simulink model "QMF_lattice"  (Simulink 7.9)
settings: Solver=ode45  StartTime=0.0  StopTime=10  RelTol=1e-3
undefined symbols (not defined in the file or in its folder): dfilt, Fs, get, sided, Two
libraries: dspsigops x6, dsparch4 x4, dspsnks4 x4, dspvision x1, simulink x1, dspsrcs4 x1
settings Model: Creator=Arun  LastModifiedBy=Arun

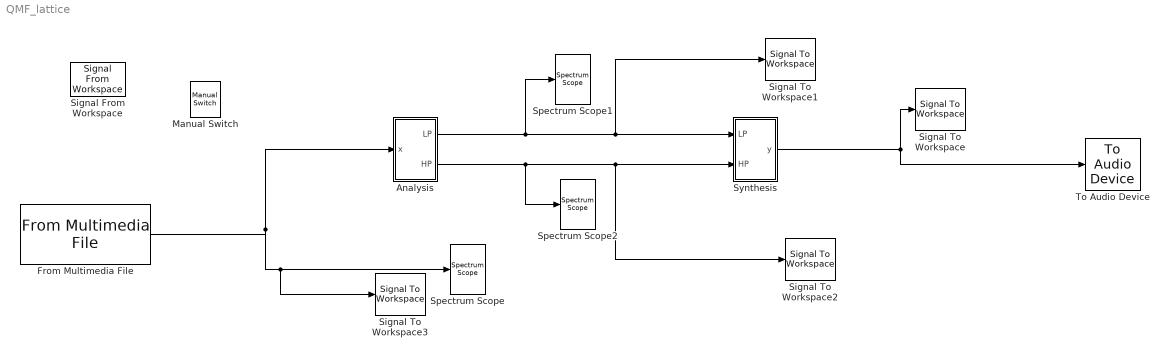
== system QMF_lattice ==
  Analysis : Subsystem
  From Multimedia File : dspvision/From Multimedia File  inputFilename=I:\Documents and Settings\Arun\My Documents\MATLAB\QMF\CRASH.WAV  loop=on  numPlays=inf  outputStreams=Audio only  videoDataType=single  audioDataType=int16  inheritSampleTime=on  userDefinedSampleTime=1/30  noAudioOutput=off  isIntensityVideo=off  fourcc=RGB  colorVideoFormat=Separate color signals  outputEOF=off  dataOrg=Column-major  audioFrameSize=1024  computeAudioFrameSize=off  outSamplingMode=Frame based
  Manual Switch : simulink/Signal Routing/Manual Switch  sw=1  action=0  varsize=off
  Signal From Workspace : dspsrcs4/Signal From Workspace  X=x  Ts=.002  nsamps=2  OutputAfterFinalValue=Setting to zero  ignoreOrWarnInputAndFrameLengths=off
  Signal To Workspace : SignalToWorkspace  VariableName=yout
      settings: CopyFcn=dspblkcopystw(gcbh);
  Signal To Workspace1 : SignalToWorkspace  VariableName=yout1
      settings: CopyFcn=dspblkcopystw(gcbh);
  Signal To Workspace2 : SignalToWorkspace  VariableName=yout2
      settings: CopyFcn=dspblkcopystw(gcbh);
  Signal To Workspace3 : SignalToWorkspace  VariableName=yout3
      settings: CopyFcn=dspblkcopystw(gcbh);
  Spectrum Scope : dspsnks4/Spectrum Scope  ScopeProperties=on  Domain=Frequency  HorizSpan=1  UseBuffer=on  BufferSize=128  Overlap=0  TreatMby1Signals=One channel  inpFftLenInherit=on  FFTlength=128  numAvg=2  DisplayProperties=off  AxisGrid=on  Memory=off  FrameNumber=on  AxisLegend=off  AxisZoom=off  OpenScopeAtSimStart=on  OpenScopeImmediately=off  FigPos=get(0,'defaultfigureposition')  AxisProperties=off  XUnits=Hertz  XRange=Two-sided ((-Fs/2...Fs/2])  XDisplay=0  InheritXIncr=on  XIncr=1.0  XLabel=Samples  XLimit=User-defined  YUnits=dBW/Hertz  XMax=11025  XMin=-11025  YLabel=Magnitude-squared, dB  LineProperties=off  wintypeSpecScope=Boxcar  RsSpecScope=50  betaSpecScope=5  winsampSpecScope=Periodic  XAxisParamsVer=6.9  isFrameUpgraded=on
      settings: YMin=6.6551  YMax=46.3833
  Spectrum Scope1 : dspsnks4/Spectrum Scope  ScopeProperties=on  Domain=Frequency  HorizSpan=1  UseBuffer=on  BufferSize=128  Overlap=0  TreatMby1Signals=One channel  inpFftLenInherit=on  FFTlength=128  numAvg=2  DisplayProperties=off  AxisGrid=on  Memory=off  FrameNumber=on  AxisLegend=off  AxisZoom=off  OpenScopeAtSimStart=on  OpenScopeImmediately=off  FigPos=get(0,'defaultfigureposition')  AxisProperties=off  XUnits=Hertz  XRange=Two-sided ((-Fs/2...Fs/2])  XDisplay=0  InheritXIncr=on  XIncr=1.0  XLabel=Samples  XLimit=User-defined  YUnits=dBW/Hertz  XMax=5512.5  XMin=-5512.5  YLabel=Magnitude-squared, dB  LineProperties=off  wintypeSpecScope=Boxcar  RsSpecScope=50  betaSpecScope=5  winsampSpecScope=Periodic  XAxisParamsVer=6.9  isFrameUpgraded=on
      settings: YMin=6.1344  YMax=52.0012
  Spectrum Scope2 : dspsnks4/Spectrum Scope  ScopeProperties=on  Domain=Frequency  HorizSpan=1  UseBuffer=on  BufferSize=128  Overlap=0  TreatMby1Signals=One channel  inpFftLenInherit=on  FFTlength=128  numAvg=2  DisplayProperties=off  AxisGrid=on  Memory=off  FrameNumber=on  AxisLegend=off  AxisZoom=off  OpenScopeAtSimStart=on  OpenScopeImmediately=off  FigPos=get(0,'defaultfigureposition')  AxisProperties=off  XUnits=Hertz  XRange=Two-sided ((-Fs/2...Fs/2])  XDisplay=0  InheritXIncr=on  XIncr=1.0  XLabel=Samples  XLimit=User-defined  YUnits=dBW/Hertz  XMax=5512.5  XMin=-5512.5  YLabel=Magnitude-squared, dB  LineProperties=off  wintypeSpecScope=Boxcar  RsSpecScope=50  betaSpecScope=5  winsampSpecScope=Periodic  XAxisParamsVer=6.9  isFrameUpgraded=on
      settings: YMin=-0.32367  YMax=44.7399
  Synthesis : Subsystem
  To Audio Device : dspsnks4/To Audio Device  deviceName=Default  inheritSampleRate=on  sampleRate=44100/2  deviceDatatype=Determine from input data type  autoBufferSize=on  bufferSize=4096  queueDuration=1.0
  wires:
  Analysis/1(LP) -> Signal To Workspace1/1, Synthesis/1(LP), Spectrum Scope1/1
  Analysis/2(HP) -> Signal To Workspace2/1, Synthesis/2(HP), Spectrum Scope2/1
  Synthesis/1(y) -> Signal To Workspace/1, To Audio Device/1
  From Multimedia File/1 -> Analysis/1(x), Spectrum Scope/1, Signal To Workspace3/1

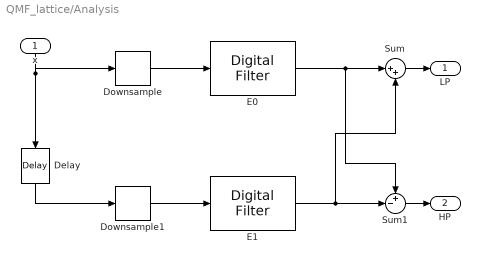
== system QMF_lattice/Analysis ==
  x : Inport
  Delay : dspsigops/Delay  InputProcessing=Columns as channels (frame based)  dly_unit=Samples  delay=1  ic_detail=off  dif_ic_for_ch=off  dif_ic_for_dly=off  ic=0  reset_popup=None
  Downsample : dspsigops/Downsample  N=2  phase=0  InputProcessing=Columns as channels (frame based)  RateOptions=Enforce single-rate processing  smode=Allow multirate  fmode=Maintain input frame size  ic=0
  Downsample1 : dspsigops/Downsample  N=2  phase=0  InputProcessing=Columns as channels (frame based)  RateOptions=Enforce single-rate processing  smode=Allow multirate  fmode=Maintain input frame size  ic=0
  E0 : dsparch4/Digital Filter  TypePopup=FIR (all zeros)  IIRFiltStruct=Direct form II transposed  AllPoleFiltStruct=Direct form  FIRFiltStruct=Direct form  CoeffSource=Specify via dialog  NumCoeffs=[ -0.006443977 ,-0.00758164 ,0.09808522 0.4807962 -0.0913825 0.02745539]  DenCoeffs=1  BiQuadCoeffs=[1 0.3 0.4 1 0.1 0.2]  LatticeCoeffs=[0.2 0.4]  denIgnore=on  FiltPerSampPopup=One filter per frame  IC=0  ICnum=0  ICden=0  roundingMode=Floor  overflowMode=off  ScaleValues=1  scaleValueFracLength=14  stageInFracLength=15  stageOutFracLength=15  FilterSource=Specify via dialog  dfiltObjectName=dfilt.dffir([1 2 1])  InputProcessing=Columns as channels (frame based)
  E1 : dsparch4/Digital Filter  TypePopup=FIR (all zeros)  IIRFiltStruct=Direct form II transposed  AllPoleFiltStruct=Direct form  FIRFiltStruct=Direct form  CoeffSource=Specify via dialog  NumCoeffs=[0.02745539 -0.0913825 0.4807962 0.09808522 -0.00758164 -0.006443977 ]  DenCoeffs=1  BiQuadCoeffs=[1 0.3 0.4 1 0.1 0.2]  LatticeCoeffs=[0.2 0.4]  denIgnore=on  FiltPerSampPopup=One filter per frame  IC=0  ICnum=0  ICden=0  roundingMode=Floor  overflowMode=off  ScaleValues=1  scaleValueFracLength=14  stageInFracLength=15  stageOutFracLength=15  FilterSource=Specify via dialog  dfiltObjectName=dfilt.dffir([1 2 1])  InputProcessing=Columns as channels (frame based)
  Sum : Sum  Inputs=|++
  Sum1 : Sum  Inputs=+-|
  LP : Outport
  HP : Outport  Port=2
  wires:
  Delay/1 -> Downsample1/1
  Downsample1/1 -> E1/1
  E0/1 -> Sum/1, Sum1/1
  E1/1 -> Sum1/2, Sum/2
  Downsample/1 -> E0/1
  x/1 -> Delay/1, Downsample/1
  Sum/1 -> LP/1
  Sum1/1 -> HP/1

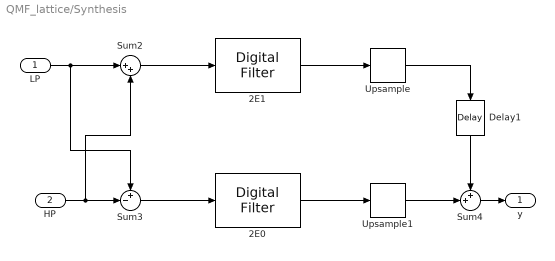
== system QMF_lattice/Synthesis ==
  LP : Inport
  HP : Inport  Port=2
  2E0 : dsparch4/Digital Filter  TypePopup=FIR (all zeros)  IIRFiltStruct=Direct form II transposed  AllPoleFiltStruct=Direct form  FIRFiltStruct=Direct form  CoeffSource=Specify via dialog  NumCoeffs=2*[ -0.006443977 ,-0.00758164 ,0.09808522 0.4807962 -0.0913825 0.02745539]  DenCoeffs=1  BiQuadCoeffs=[1 0.3 0.4 1 0.1 0.2]  LatticeCoeffs=[0.2 0.4]  denIgnore=on  FiltPerSampPopup=One filter per frame  IC=0  ICnum=0  ICden=0  roundingMode=Floor  overflowMode=off  ScaleValues=1  scaleValueFracLength=14  stageInFracLength=15  stageOutFracLength=15  FilterSource=Specify via dialog  dfiltObjectName=dfilt.dffir([1 2 1])  InputProcessing=Columns as channels (frame based)
  2E1 : dsparch4/Digital Filter  TypePopup=FIR (all zeros)  IIRFiltStruct=Direct form II transposed  AllPoleFiltStruct=Direct form  FIRFiltStruct=Direct form  CoeffSource=Specify via dialog  NumCoeffs=2*[0.02745539 -0.0913825 0.4807962 0.09808522 -0.00758164 -0.006443977 ]  DenCoeffs=1  BiQuadCoeffs=[1 0.3 0.4 1 0.1 0.2]  LatticeCoeffs=[0.2 0.4]  denIgnore=on  FiltPerSampPopup=One filter per frame  IC=0  ICnum=0  ICden=0  roundingMode=Floor  overflowMode=off  ScaleValues=1  scaleValueFracLength=14  stageInFracLength=15  stageOutFracLength=15  FilterSource=Specify via dialog  dfiltObjectName=dfilt.dffir([1 2 1])  InputProcessing=Columns as channels (frame based)
  Delay1 : dspsigops/Delay  InputProcessing=Columns as channels (frame based)  dly_unit=Samples  delay=1  ic_detail=off  dif_ic_for_ch=off  dif_ic_for_dly=off  ic=0  reset_popup=None
  Sum2 : Sum  Inputs=|++
  Sum3 : Sum  Inputs=+-|
  Sum4 : Sum  Inputs=++|
  Upsample : dspsigops/Upsample  N=2  phase=0  InputProcessing=Columns as channels (frame based)  RateOptions=Enforce single-rate processing  ic=0  mode=Unused parameter value
  Upsample1 : dspsigops/Upsample  N=2  phase=0  InputProcessing=Columns as channels (frame based)  RateOptions=Enforce single-rate processing  ic=0  mode=Unused parameter value
  y : Outport
  wires:
  LP/1 -> Sum2/1, Sum3/1
  Sum2/1 -> 2E1/1
  HP/1 -> Sum2/2, Sum3/2
  Sum3/1 -> 2E0/1
  2E0/1 -> Upsample1/1
  2E1/1 -> Upsample/1
  Upsample/1 -> Delay1/1
  Delay1/1 -> Sum4/1
  Upsample1/1 -> Sum4/2
  Sum4/1 -> y/1
